simulink model "PosControl_HIL_advanced"  (R2023b)
settings: Solver=FixedStepDiscrete  StartTime=0.0  StopTime=10.0  FixedStep=0.001  RelTol=1e-3
InitFcn:
  | Init_control
values from neighbouring files (symbols this model uses):
  DEG2RAD = 0.0174533    [Init_control.m]
  MAX_CONTROL_ANGLE_RATE_PITCH = 220    [Init_control.m]
  MAX_CONTROL_ANGLE_RATE_ROLL = 220    [Init_control.m]
  MAX_CONTROL_VELOCITY_XY = 5    [Init_control.m]
  MAX_CONTROL_VELOCITY_Z = 3    [Init_control.m]
  Saturation_I_az = 5    [Init_control.m]
undefined symbols (not defined in the file or in its folder): DiscIntNeverNeededParam
libraries: simulink x7, pixhawk_slib_uORB_RW x5, pixhawk_slib_sensors_actuators x4
(part 2 of 2)

== matlab function PosControl_HIL_advanced/Control System/pwm_out2 ==
  data: Roll input; M1 output; Pitch input; Yaw input; Thrust input; M2 output; M3 output; M4 output; Kill input; arm_com input; resti input; vze input
function [M1, M2, M3, M4] = motor_mixer(Roll,Pitch,Yaw,Thrust,Kill,arm_com, resti, vze)
%Function description:
%  Control allocation. The quadrotor type is X-configuration,
%  and the airframe is as follows:
%3↓   1↑
 %  \ /
 %  / \
 %2↑   4↓
%Input：
%  Roll, Pitch, Yaw: attitude controller output.
%  Thrust

idle_PWM = 1100;
scale = 2000 - idle_PWM;

if arm_com > 0.5  % 锁定,  1：解锁，0：锁定
    M1 = (Thrust - Roll + Pitch + Yaw) * scale + idle_PWM;
    M2 = (Thrust + Roll - Pitch + Yaw) * scale + idle_PWM;
    M3 = (Thrust + Roll + Pitch - Yaw) * scale + idle_PWM;
    M4 = (Thrust - Roll - Pitch - Yaw) * scale + idle_PWM;
else
    M1 = 900;
    M2 = 900;
    M3 = 900;
    M4 = 900;
end

if (Kill<1.5 && Kill>0.5) % 3为正常  % 1为Kill，如果QGC没有指定Kill，则Kill=0
    M1 = 900;
    M2 = 900;
    M3 = 900;
    M4 = 900;
end

== matlab function PosControl_HIL_advanced/MATLAB Function1 ==
  data: XX_read input; XX output
function XX = fcn(XX_read)
if isnan(XX_read) 
    XX = 0;
else
    XX = XX_read;
end
